simulink model "BiT_Template"  (R2024b)
settings: Solver=FixedStepDiscrete  StartTime=0.0  StopTime=Inf  FixedStep=0.005  RelTol=1e-3
StopFcn:
  | user_confirmed = true;
  | disp('Gestoppt?!')
  | 
  | % stop(t);
  | % delete(t);
  | 
  | %% Switch to Config Mode
  | %Tc3_AI.sysManager.ActivateConfiguration();
  | %
  | % Tc3_AI.SwitchToConfig('local')
  | %
  | % %save Solution
  | % Tc3_AI.SaveSolution();
  | %
  | % %% Close Aktive VS Instance
  | % Tc3_AI.closeVsInstance();
libraries: slpidlib x1
settings Model: SimulationMode=external  Creator=clemensm  LastModifiedBy=pikronthaler
settings OptimizationCC: LocalBlockOutputs=off
settings RTWCC: Description=TwinCAT GRT Target  SystemTargetFile=TwinCatGrt.tlc  GenCodeOnly=on  GenerateMakefile=off  TemplateMakefile=tcgrt_msbuild.tmf  TargetLang=C++
settings STFCustomTargetCC: TargetLangStandard=C++11 (ISO)  ConcurrentExecutionCompliant=on  CombineOutputUpdateFcns=on  CodeInterfacePackaging=Reusable function  CPPClassGenCompliant=on  GenerateAllocFcn=on  SystemTargetFile=TwinCatGrt.tlc
settings GRTTargetCC: TargetLangStandard=C++11 (ISO)  ParMdlRefBuildCompliant=off  CompOptLevelCompliant=off  MatFileLogging=off  CodeInterfacePackaging=Reusable function  GenerateAllocFcn=on  UseToolchainInfoCompliant=off  ExtMode=on  ExtModeMexFile=TcExtModeClient  MultiInstanceErrorCode=None

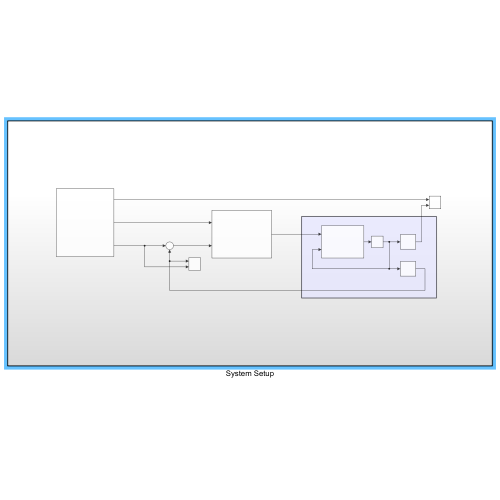
[thumbnail: Simulink's stored preview of the top-level diagram]
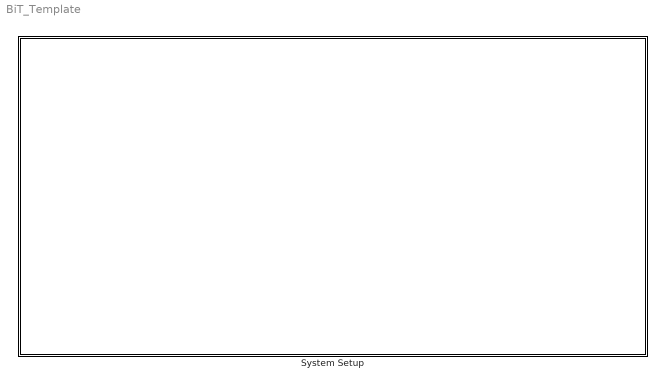
== system BiT_Template ==
  System Setup : Subsystem

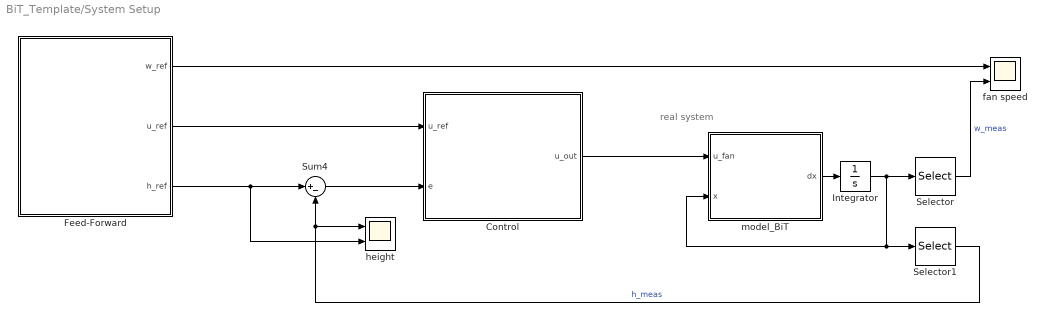
== system BiT_Template/System Setup ==
  note: real system
  Control : Subsystem
  Feed-Forward : Subsystem
  Integrator : Integrator
  Selector : Selector  InputPortWidth=3  IndexOptions=Index vector (dialog)  Indices=3  OutputSizes=1
  Selector1 : Selector  InputPortWidth=3  IndexOptions=Index vector (dialog)  Indices=1  OutputSizes=1
  Sum4 : Sum  Inputs=|+-
  fan speed : Scope  NumInputPorts=2
  height : Scope  NumInputPorts=2
  model_BiT : MATLAB Function  TreatAsAtomicUnit=on
  wires:
  Selector1/1 -> height/1, Sum4/2  "h_meas"
  Selector/1 -> fan speed/2  "w_meas"
  model_BiT/1(dx) -> Integrator/1
  Integrator/1 -> Selector/1, Selector1/1, model_BiT/2(x)
  Feed-Forward/3(h_ref) -> height/2, Sum4/1
  Feed-Forward/1(w_ref) -> fan speed/1
  Feed-Forward/2(u_ref) -> Control/1(u_ref)
  Sum4/1 -> Control/2(e)
  Control/1(u_out) -> model_BiT/1(u_fan)

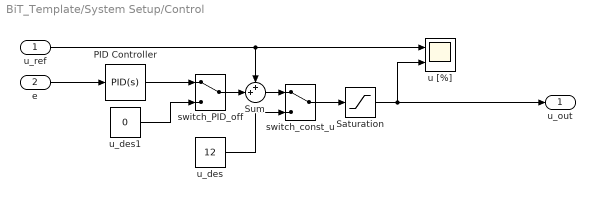
== system BiT_Template/System Setup/Control ==
  u_ref : Inport
  e : Inport  Port=2
  PID Controller : slpidlib/PID Controller  Controller=PID  Form=Parallel  TimeDomain=Continuous-time  UseExternalTs=off  SampleTime=-1  IntegratorMethod=Forward Euler  FilterMethod=Forward Euler  ControllerParametersSource=internal  P=1  I=1  UseKiTs=off  D=0  UseExternalDerivativeSource=off  N=100  UseFilter=on  TunerSelectOption=Transfer Function Based (PID Tuner App)  InitialConditionSource=internal  InitialConditionForIntegrator=0  InitialConditionForFilter=0  DifferentiatorICPrevScaledInput=0  ExternalReset=none  TrackingMode=off  Kt=1  LimitOutput=off  SatLimitsSource=internal  UpperSaturationLimit=inf  LowerSaturationLimit=-inf  LinearizeAsGain=on  AntiWindupMode=none  Kb=1  LimitIntegrator=off  UpperIntegratorSaturationLimit=inf  LowerIntegratorSaturationLimit=-inf  POutMin=[]  POutMax=[]  IOutMin=[]  IOutMax=[]  DOutMin=[]  DOutMax=[]  NOutMin=[]  NOutMax=[]  SumOutMin=[]  SumOutMax=[]  SaturationOutMin=[]  SaturationOutMax=[]  PParamMin=[]  PParamMax=[]  IParamMin=[]  IParamMax=[]  DParamMin=[]  DParamMax=[]  NParamMin=[]  NParamMax=[]  KbParamMin=[]  KbParamMax=[]  KtParamMin=[]  KtParamMax=[]  KbOutMin=[]  KbOutMax=[]  KtOutMin=[]  KtOutMax=[]  IntegratorOutMin=[]  IntegratorOutMax=[]  FilterOutMin=[]  FilterOutMax=[]  SumI1OutMin=[]  SumI1OutMax=[]  SumI2OutMin=[]  SumI2OutMax=[]  SumI3OutMin=[]  SumI3OutMax=[]  SumI4OutMin=[]  SumI4OutMax=[]  SumDOutMin=[]  SumDOutMax=[]  DifferentiatorOutMin=[]  DifferentiatorOutMax=[]  FilterDiffOutCoefMin=[]  FilterDiffOutCoefMax=[]  ReciprocalOutMin=[]  ReciprocalOutMax=[]  SumDenOutMin=[]  SumDenOutMax=[]  SumNumOutMin=[]  SumNumOutMax=[]  DivideOutMin=[]  DivideOutMax=[]  UdiffTsProdOutMin=[]  UdiffTsProdOutMax=[]  NTsProdOutMin=[]  NTsProdOutMax=[]  UintegralTsProdOutMin=[]  UintegralTsProdOutMax=[]  UngainTsProdOutMin=[]  UngainTsProdOutMax=[]  ClampingZeroOutDataTypeStr=Inherit: Inherit via back propagation  ClampingZeroOutMin=[]  ClampingZeroOutMax=[]  FilterDenConstantOutDataTypeStr=Inherit: Inherit via back propagation  FilterDenConstantOutMin=[]  FilterDenConstantOutMax=[]  PCopyOutDataTypeStr=Inherit: Inherit via back propagation  PCopyOutMin=[]  PCopyOutMax=[]  NCopyOutDataTypeStr=Inherit: Inherit via back propagation  NCopyOutMin=[]  NCopyOutMax=[]  IntegratorContinuousStateAttributes=''  IntegratorStateMustResolveToSignalObject=off  IntegratorRTWStateStorageClass=Auto  FilterContinuousStateAttributes=''  FilterStateMustResolveToSignalObject=off  FilterRTWStateStorageClass=Auto  ParallelPVariant=InternalParameters  IdealPVariant=Disabled  IVariant=InternalParameters  DVariant=InternalParameters  IntegratorVariant=Continuous  SatVariant=Disabled  AWVariant=Passthrough  PCopyVariant=Disabled  TRVariant=Disabled  FdbkBlocksVariant=Forward  IdealPFdbkVariant=Disabled  SatFdbkVariant=Disabled  DerivativeFilterVariant=ContFilter  NVariant=InternalParameters  NCopyVariant=Disabled  FilterICVariant=InternalICsFilter  IntegratorICVariant=InternalICs  ExternalResetVariant=Disabled  TRSumVariant=Passthrough  SumFdbkVariant=Disabled  SumVariant=Sum_PID  TsampFilterVariant=InternalTs  TsampNgainVariant=Passthrough  TsampIntegralVariant=Passthrough  ExternalSaturationOutDataTypeStr=Inherit: Same as second input  DerivativeSourceVariant=ErrorSignal  PreIntVariant=InternalPreInt
  Saturation : Saturate  UpperLimit=100  LowerLimit=0
  Sum : Sum  Inputs=++|
  switch_PID_off : ManualSwitch
  switch_const_u : ManualSwitch
  u [%] : Scope  NumInputPorts=2
  u_des : Constant  Value=12
  u_des1 : Constant  Value=0
  u_out : Outport
  wires:
  u_des/1 -> switch_const_u/2
  Saturation/1 -> u_out/1, u [%]/2
  e/1 -> PID Controller/1
  switch_const_u/1 -> Saturation/1
  u_ref/1 -> u [%]/1, Sum/1
  Sum/1 -> switch_const_u/1
  PID Controller/1 -> switch_PID_off/1
  switch_PID_off/1 -> Sum/2
  u_des1/1 -> switch_PID_off/2

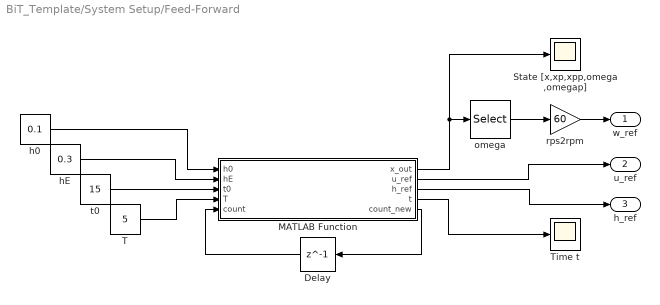
== system BiT_Template/System Setup/Feed-Forward ==
  Delay : Delay  DelayLength=1
  MATLAB Function : MATLAB Function  TreatAsAtomicUnit=on
  State [x,xp,xpp,omega,omegap] : Scope
  T : Constant  Value=5
  Time t : Scope
  h0 : Constant  Value=0.1
  hE : Constant  Value=0.3
  omega : Selector  InputPortWidth=5  IndexOptions=Index vector (dialog)  Indices=4  OutputSizes=1
  rps2rpm : Gain  Gain=60
  t0 : Constant  Value=15
  w_ref : Outport
  u_ref : Outport  Port=2
  h_ref : Outport  Port=3
  wires:
  h0/1 -> MATLAB Function/1(h0)
  omega/1 -> rps2rpm/1
  MATLAB Function/4(t) -> Time t/1
  T/1 -> MATLAB Function/4(T)
  t0/1 -> MATLAB Function/3(t0)
  Delay/1 -> MATLAB Function/5(count)
  MATLAB Function/5(count_new) -> Delay/1
  hE/1 -> MATLAB Function/2(hE)
  MATLAB Function/1(x_out) -> State [x,xp,xpp,omega,omegap]/1, omega/1
  MATLAB Function/2(u_ref) -> u_ref/1
  MATLAB Function/3(h_ref) -> h_ref/1
  rps2rpm/1 -> w_ref/1

== matlab function BiT_Template/System Setup/model_BiT ==
  data: u_fan input; dx output; x input
function dx  = model_BiT(u_fan,x)
% model_BiT represents the differential equations of the ball in tube test
% rig

% u_fan ... duty cycle in [%]
% x[3] ... state that includes
%       x1 = h ... height of the ball in [m]
%       x2 = dh ... change of heihgt of the ball in [m/s]
%       x3 = w ... fan speed in [rpm]


dx = zeros(3,1);

== matlab function BiT_Template/System Setup/Feed-Forward/MATLAB Function ==
  data: x_out output; u_ref output; h0 input; hE input; t0 input; T input; h_ref output; t output; count input; count_new output
function [x_out,u_ref,h_ref,t,count_new] = feed_forward(h0,hE,t0,T,count)

count_new = count+1;
dT = 0.005;
t = count_new*dT-t0;

% Parameter



% Calculate Trajectory

xp_ref = 0;
xpp_ref = 0;
xppp_ref = 0;

if t<0
    x_ref = h0;
elseif t>T
    x_ref = hE;
else
    x_ref = h0; % Trajectory has to be implemented!
end

% Equations:
omega = 0; % equation for omega
omega_p = 0; % equation for omega
u = 0; % equation for omega

h_ref = x_ref;
u_ref = u; 
x_out = [x_ref,xp_ref,xpp_ref,omega,omega_p]';
end
